simulink model "MRAS_IR2_Ld_Lq"  (R2019b)
settings: Solver=ode23tb  StartTime=0.0  StopTime=3  MaxStep=1e-5  RelTol=5e-4  EnableMultiTasking=on
libraries: powerlib x8, powerlib_meascontrol x2, simulink x1
settings Model: Creator=Алексей  LastModifiedBy=Len_comp
settings SolverCC: ZeroCrossControl=DisableAll  ZeroCrossAlgorithm=Adaptive
settings DataIOCC: SaveFormat=Array  SaveOutput=off  DSMLogging=off  SaveTime=off  ReturnWorkspaceOutputs=off
settings OptimizationCC: LifeSpan=inf
settings DebuggingCC: UnderspecifiedInitializationDetection=Classic  MergeDetectMultiDrivingBlocksExec=none  SolverPrmCheckMsg=warning  AllowSymbolicDim=off  SFUnexpectedBacktrackingDiag=warning  SFNoUnconditionalDefaultTransitionDiag=warning  SFExecutionAtInitializationDiag=none  ArithmeticOperatorsInVariantConditions=warning
settings HardwareCC: ProdBitPerPointer=32  ProdBitPerSizeT=32  ProdBitPerPtrDiffT=32  ProdLargestAtomicFloat=None  ProdIntDivRoundTo=Undefined  ProdEndianess=Unspecified  ProdWordSize=32  ProdHWDeviceType=32-bit Generic
settings ModelReferenceCC: PropagateSignalLabelsOutOfModel=off
settings SFSimCC: SimUseLocalCustomCode=off  CustomCodeUndefinedFunction=UseInterfaceOnly
settings RTWCC: RTWUseLocalCustomCode=off
settings CodeAppCC: StateflowObjectComments=on
settings GRTTargetCC: TargetLangStandard=C89/C90 (ANSI)  GeneratePreprocessorConditionals=Disable all
settings ConfigComp: CovMetricSettings=dw  CovHtmlReporting=on  CovSaveCumulativeToWorkspaceVar=on  CovSaveSingleToWorkspaceVar=on  CovExternalEMLEnable=off  CovSFcnEnable=off
settings SimscapeCC: SimscapeNormalizeSystem=off

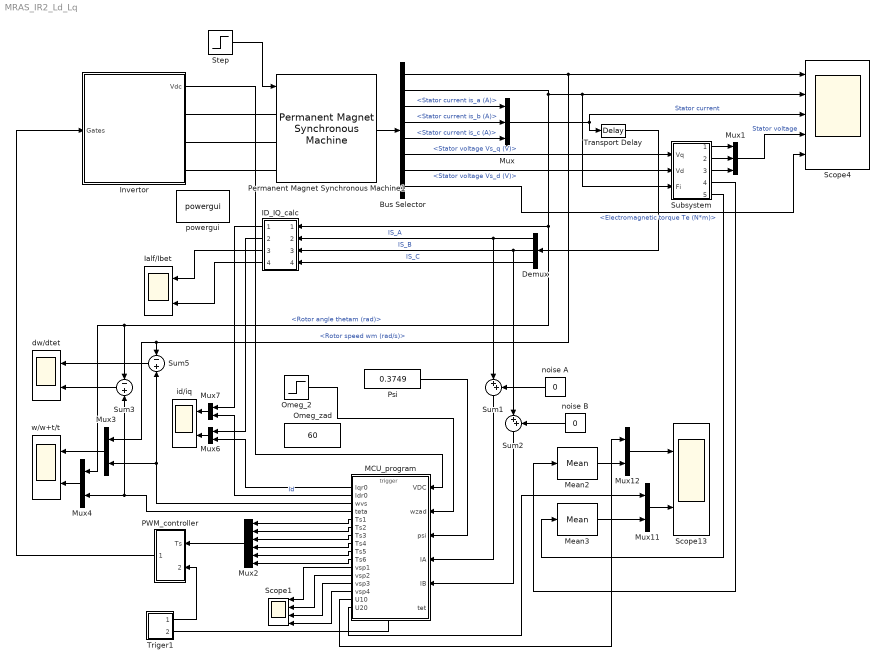
== system MRAS_IR2_Ld_Lq ==
  Bus Selector : BusSelector  OutputSignals=Rotor speed wm (rad/s),Rotor angle thetam (rad),Stator current is_a (A),Stator current is_b (A),Stator current is_c (A),Stator voltage Vs_q (V),Stator voltage Vs_d (V),Electromagnetic torque Te (N*m)
  Demux : Demux  Outputs=3
  ID_IQ_calc : Subsystem
  Ialf/Ibet : Scope  NumInputPorts=2
  Invertor : Subsystem
  MCU_program : MATLAB Function  TreatAsAtomicUnit=on
  Mean2 : powerlib_meascontrol/Measurements/Mean  Freq=10000  Vinit=0  Ts=0
      settings: SourceProductName=Simscape Electrical
  Mean3 : powerlib_meascontrol/Measurements/Mean  Freq=10000  Vinit=0  Ts=0
      settings: SourceProductName=Simscape Electrical
  Mux : Mux  Inputs=3
  Mux1 : Mux  Inputs=3
  Mux{3..4,6..7,11..12} (6 alike) : Mux  Inputs=2
  Mux2 : Mux  Inputs=6
  Omeg_2 : Step  Time=2.4  Before=60  After=100  SampleTime=0
  Omeg_zad : Constant  Value=60
  PWM_controller : Subsystem
  Permanent Magnet Synchronous Machine1 : powerlib/Machines/Permanent Magnet Synchronous Machine  NbPhases=3  FluxDistribution=Sinusoidal  RotorType=Salient-pole  MechanicalLoad=Torque Tm  PresetModel=No  ShowDetailedParameters=on  MeasurementBus=off  Resistance=13.75  Inductance=8.5e-3  dqInductances=[44e-3,39.8e-3]  La=40e-3  MachineConstant=Voltage Constant (V_peak L-L / krpm)  Flux=0.3749  VoltageCst=68  TorqueCst=0.56236  Flat=120  Mechanical=[2e-04 3e-03 1 0]  PolePairs=1  InitialConditions=[0,0, 0,0]  InitialConditions5ph=[0 0 0 0 0 0]  RefAngle=Aligned with phase A axis (original Park)  IterativeDiscreteModel=Trapezoidal non iterative  TsBlock=-1  TsPowergui=0
  Psi : Constant  Value=0.3749
  Scope1 : Scope  NumInputPorts=4
  Scope13 : Scope  NumInputPorts=2
  Scope4 : Scope  NumInputPorts=5
  Step : Step  Time=1.8  Before=0.02  After=0.07  SampleTime=0
  Subsystem : Subsystem
  Sum1 : Sum  Inputs=|++
  Sum2 : Sum  Inputs=|++
  Sum3 : Sum  Inputs=-+
  Sum5 : Sum  Inputs=-+
  Transport Delay : TransportDelay  DelayTime=5e-6
  Triger1 : Subsystem
  dw/dtet : Scope  NumInputPorts=2
  id/iq : Scope  NumInputPorts=2
  noise A : Constant  Value=0
  noise B : Constant  Value=0
  powergui : powerlib/powergui  Priority=1  SimulationMode=Continuous  SampleTime=50e-6  frequency=60  Iterations=50  frequencyindice=0  Pbase=100e6  ErrMax=1e-4  UnitsV=kV  UnitsW=MW  buscounter=0  FunctionMessages=off  echomessages=off  EnableUseOfTLC=off  CurrentSourceSwitches=on  DisableSnubberDevices=off  DisableRonSwitches=off  DisableVfSwitches=off  DisplayEquations=off  AutomaticDiscreteSolvers=off  SolverType=Tustin  Interpol=off  ExternalGateDelay=off  methode=off  Ts=0  x0status=blocks  SPID=off  SwTol=0  HookPort=off  NonlinearTolerance=1e-4  nMaxIteration=100  ContinueOnMaxIteration=off  RestoreLinks=warning  ResistiveCurrentMeasurement=off  Frange=[0:2:500]  Ylog=off  Xlog=on  ShowGrid=off  save=off  variable=ZData  structure=SD2  ZoomFFT=on  StartTime=0.7  cycles=10  DisplayStyle=4  fundamental=382  FreqAxis=off  MaxFrequency=50000  frequencyindicesteady=1  RmsSteady=1  display=off
      settings: SourceProductName=Simscape Electrical
  w/w+t/t : Scope  NumInputPorts=2
  wires:
  Demux/1 -> ID_IQ_calc/2(In2), Sum1/1  "IS_A"
  Demux/2 -> ID_IQ_calc/3(In3), Sum2/1  "IS_B"
  MCU_program/2(Idr0) -> Mux7/2  "Id"
  Omeg_2/1 -> MCU_program/2(wzad)
  Permanent Magnet Synchronous Machine1/1 -> Bus Selector/1
  Bus Selector/3 -> Mux/1  "<Stator current is_a (A)>"
  Bus Selector/4 -> Mux/2  "<Stator current is_b (A)>"
  Bus Selector/5 -> Mux/3  "<Stator current is_c (A)>"
  Bus Selector/6 -> Subsystem/1(Vq)  "<Stator voltage Vs_q (V)>"
  Bus Selector/7 -> Subsystem/2(Vd)  "<Stator voltage Vs_d (V)>"
  Subsystem/2(Out2) -> Mux1/2
  Subsystem/3(Out3) -> Mux1/3
  Subsystem/1(Out1) -> Mux1/1
  Mux/1 -> Scope4/3, Transport Delay/1  "Stator current"
  MCU_program/3(wvs) -> Mux3/2, Sum5/2
  Mux1/1 -> Scope4/4  "Stator voltage"
  Bus Selector/8 -> Scope4/5  "<Electromagnetic torque Te (N*m)>"
  Mux7/1 -> id/iq/1
  Mux6/1 -> id/iq/2
  Demux/3 -> ID_IQ_calc/4(In4)  "IS_C"
  Sum3/1 -> dw/dtet/2
  Sum5/1 -> dw/dtet/1
  MCU_program/4(teta) -> Mux4/2, Sum3/2
  ID_IQ_calc/1(Out1) -> Mux7/1
  ID_IQ_calc/2(Out2) -> Mux6/1
  Step/1 -> Permanent Magnet Synchronous Machine1/1
  MCU_program/5(Ts1) -> Mux2/1
  MCU_program/6(Ts2) -> Mux2/2
  MCU_program/7(Ts3) -> Mux2/3
  MCU_program/8(Ts4) -> Mux2/4
  MCU_program/9(Ts5) -> Mux2/5
  MCU_program/10(Ts6) -> Mux2/6
  Mux2/1 -> PWM_controller/1(Ts)
  Triger1/1(1) -> PWM_controller/2(pila)
  PWM_controller/1(Tss) -> Invertor/1(Gates)
  Mux3/1 -> w/w+t/t/1
  Mux4/1 -> w/w+t/t/2
  MCU_program/12(vsp2) -> Scope1/2
  MCU_program/13(vsp3) -> Scope1/3
  MCU_program/11(vsp1) -> Scope1/1
  Sum1/1 -> MCU_program/4(IA)
  Sum2/1 -> MCU_program/5(IB)
  Psi/1 -> MCU_program/3(psi)
  MCU_program/15(U10) -> Mux12/1
  Bus Selector/1 -> Scope4/1, Mux3/1, Sum5/1  "<Rotor speed wm (rad/s)>"
  Bus Selector/2 -> Mux4/1, Sum3/1, ID_IQ_calc/1(In1), Scope4/2, Subsystem/3(Fi)  "<Rotor angle thetam (rad)>"
  Triger1/2(2) -> MCU_program/Trigger
  MCU_program/16(U20) -> Mux11/1
  Mux12/1 -> Scope13/1
  Mux11/1 -> Scope13/2
  Mean3/1 -> Mux11/2
  Mean2/1 -> Mux12/2
  Invertor/1(Vdc) -> MCU_program/1(VDC)
  Subsystem/4(Out4) -> Mean2/1
  Subsystem/5(Out5) -> Mean3/1
  Transport Delay/1 -> Demux/1
  MCU_program/1(Iqr0) -> Mux6/2
  noise A/1 -> Sum1/2
  noise B/1 -> Sum2/2
  MCU_program/14(vsp4) -> Scope1/4
  ID_IQ_calc/3(Out3) -> Ialf/Ibet/1
  ID_IQ_calc/4(Out4) -> Ialf/Ibet/2
  connections:
  Permanent Magnet Synchronous Machine1/LConn1 -- Invertor/RConn1
  Invertor/RConn3 -- Permanent Magnet Synchronous Machine1/LConn3
  Permanent Magnet Synchronous Machine1/LConn2 -- Invertor/RConn2

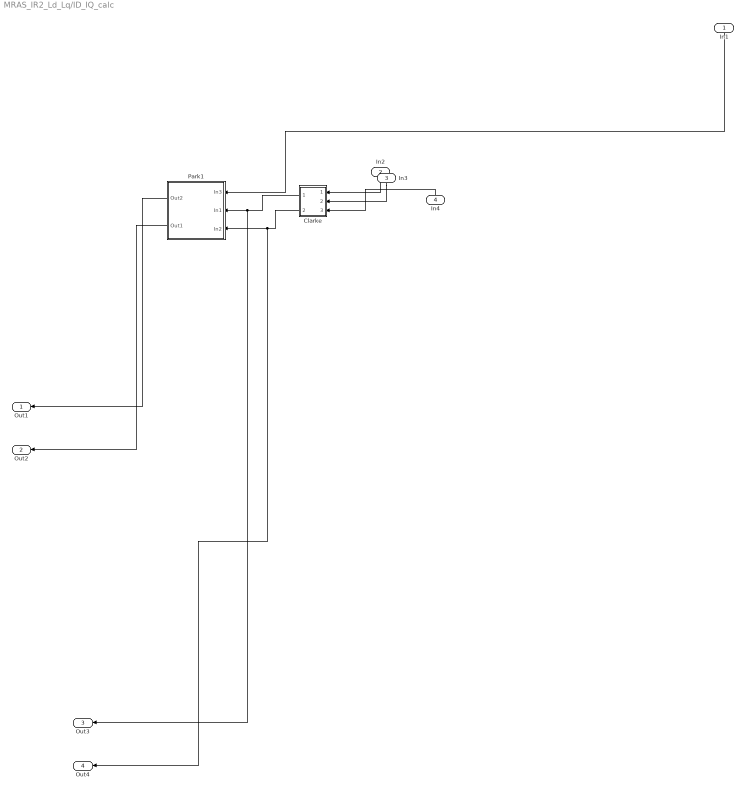
== system MRAS_IR2_Ld_Lq/ID_IQ_calc ==
  In1 : Inport
  In2 : Inport  Port=2
  In3 : Inport  Port=3
  In4 : Inport  Port=4
  Clarke : Subsystem
  Park1 : Subsystem
  Out1 : Outport
  Out2 : Outport  Port=2
  Out3 : Outport  Port=3
  Out4 : Outport  Port=4
  wires:
  Park1/2(Out1) -> Out2/1
  Park1/1(Out2) -> Out1/1
  In1/1 -> Park1/1(In3)
  In4/1 -> Clarke/3(In3)
  In2/1 -> Clarke/1(In1)
  In3/1 -> Clarke/2(In2)
  Clarke/2(Out1) -> Out4/1, Park1/3(In2)
  Clarke/1(Out2) -> Out3/1, Park1/2(In1)

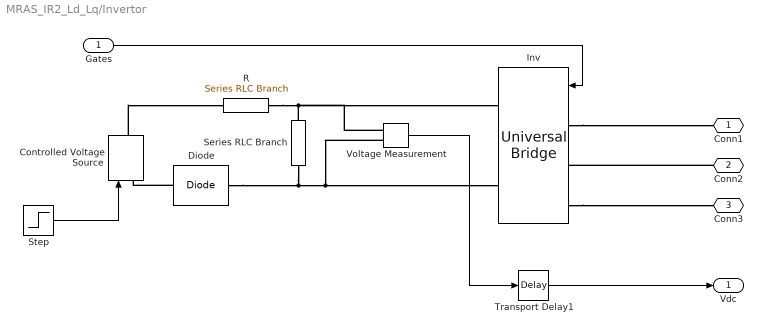
== system MRAS_IR2_Ld_Lq/Invertor ==
  Gates : Inport
  Controlled Voltage Source : powerlib/Electrical Sources/Controlled Voltage Source  Initialize=on  Source_Type=AC  Amplitude=0  Phase=0  Frequency=0  Measurements=None
      settings: SourceProductName=Simscape Electrical
  Diode : powerlib/Power Electronics/Diode  Ron=0.001  Lon=0  Vf=0.8  IC=0  UseSnubber=off  Rs=500  Cs=250e-9  Measurements=off
      settings: SourceProductName=Simscape Electrical
  Inv : powerlib/Power Electronics/Universal Bridge  Arms=3  SnubberResistance=1e5  SnubberCapacitance=inf  Device=IGBT / Diodes  Ron=1e-3  Lon=0  ForwardVoltages="[  3  3  ]"  ForwardVoltage=0  GTOparameters=[ 10e-6 , 20e-6 ]  IGBTparameters=[ 1e-7 , 2e-7 ]  Measurements=UAB UBC UCA UDC voltages  Measurements_2=None  converterType=Rectifier
      settings: SourceProductName=Simscape Electrical
  R : powerlib/Elements/Series RLC Branch  LConnTagsString=__new0  RConnTagsString=__new0  BranchType=R  Resistance=0.01  Inductance=1e-3  SetiL0=off  InitialCurrent=0  Capacitance=30e-6  Setx0=on  InitialVoltage=220  Measurements=None
      settings: SourceProductName=Simscape Electrical
  Series RLC Branch : powerlib/Elements/Series RLC Branch  LConnTagsString=__new0  RConnTagsString=__new0  BranchType=C  Resistance=1  Inductance=1e-3  SetiL0=off  InitialCurrent=0  Capacitance=30e-6  Setx0=on  InitialVoltage=20  Measurements=None
      settings: SourceProductName=Simscape Electrical
  Step : Step  Time=5.06  Before=150  After=300  SampleTime=0
  Transport Delay1 : TransportDelay  DelayTime=26e-6
  Voltage Measurement : powerlib/Measurements/Voltage Measurement  PhasorSimulation=off  OutputType=Complex  PSBequivalent=0
      settings: SourceProductName=Simscape Electrical
  Conn1 : PMIOPort  Side=Right
  Conn2 : PMIOPort  Port=2  Side=Right
  Conn3 : PMIOPort  Port=3  Side=Right
  Vdc : Outport
  wires:
  Gates/1 -> Inv/1
  Voltage Measurement/1 -> Transport Delay1/1
  Transport Delay1/1 -> Vdc/1
  Step/1 -> Controlled Voltage Source/1
  connections:
  Diode/LConn1 -- Series RLC Branch/RConn1 -- Voltage Measurement/LConn2 -- Inv/RConn2
  Series RLC Branch/LConn1 -- Voltage Measurement/LConn1 -- Inv/RConn1 -- R/LConn1
  Conn2/RConn1 -- Inv/LConn2
  Diode/RConn1 -- Controlled Voltage Source/LConn1
  Inv/LConn3 -- Conn3/RConn1
  Inv/LConn1 -- Conn1/RConn1
  Controlled Voltage Source/RConn1 -- R/RConn1

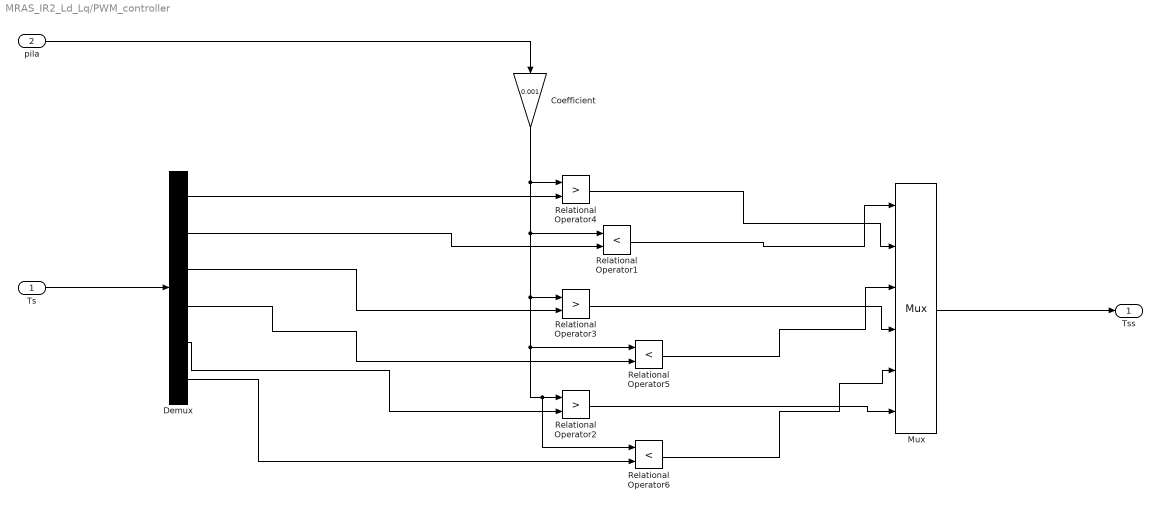
== system MRAS_IR2_Ld_Lq/PWM_controller ==
  Ts : Inport
  pila : Inport  Port=2
  Coefficient : Gain  Gain=0.001
  Demux : Demux  Outputs=6
  Mux : Mux  Inputs=6
  Relational Operator1 : RelationalOperator  Operator=<  OutDataTypeStr=boolean  RndMeth=Nearest
  Relational Operator2 : RelationalOperator  Operator=>  OutDataTypeStr=boolean  RndMeth=Nearest
  Relational Operator3 : RelationalOperator  Operator=>  OutDataTypeStr=boolean  RndMeth=Nearest
  Relational Operator4 : RelationalOperator  Operator=>  OutDataTypeStr=boolean  RndMeth=Nearest
  Relational Operator5 : RelationalOperator  Operator=<  OutDataTypeStr=boolean  RndMeth=Nearest
  Relational Operator6 : RelationalOperator  Operator=<  OutDataTypeStr=boolean  RndMeth=Nearest
  Tss : Outport
  wires:
  Relational Operator4/1 -> Mux/2
  Demux/3 -> Relational Operator3/2
  Demux/5 -> Relational Operator2/2
  Relational Operator3/1 -> Mux/4
  Relational Operator2/1 -> Mux/6
  Ts/1 -> Demux/1
  Coefficient/1 -> Relational Operator1/1, Relational Operator3/1, Relational Operator5/1, Relational Operator6/1, Relational Operator2/1, Relational Operator4/1
  Relational Operator1/1 -> Mux/1
  Relational Operator5/1 -> Mux/3
  Relational Operator6/1 -> Mux/5
  Demux/2 -> Relational Operator1/2
  Demux/4 -> Relational Operator5/2
  Demux/6 -> Relational Operator6/2
  Demux/1 -> Relational Operator4/2
  pila/1 -> Coefficient/1
  Mux/1 -> Tss/1

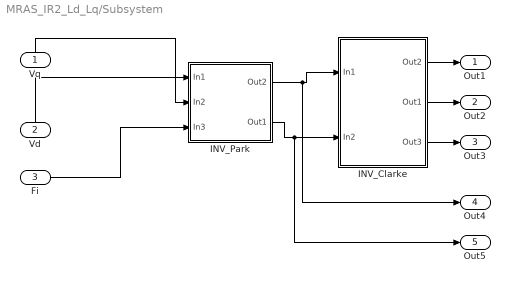
== system MRAS_IR2_Ld_Lq/Subsystem ==
  Vq : Inport
  Vd : Inport  Port=2
  Fi : Inport  Port=3
  INV_Clarke : Subsystem
  INV_Park : Subsystem
  Out1 : Outport
  Out2 : Outport  Port=2
  Out3 : Outport  Port=3
  Out4 : Outport  Port=4
  Out5 : Outport  Port=5
  wires:
  INV_Clarke/2(Out1) -> Out2/1
  INV_Park/1(Out2) -> Out4/1, INV_Clarke/1(In1)
  INV_Clarke/1(Out2) -> Out1/1
  INV_Park/2(Out1) -> Out5/1, INV_Clarke/2(In2)
  INV_Clarke/3(Out3) -> Out3/1
  Fi/1 -> INV_Park/3(In3)
  Vd/1 -> INV_Park/1(In1)
  Vq/1 -> INV_Park/2(In2)

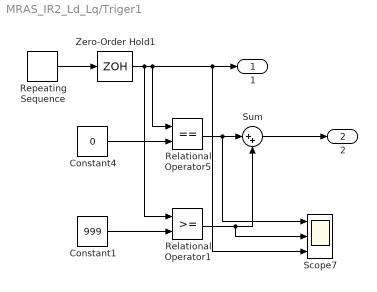
== system MRAS_IR2_Ld_Lq/Triger1 ==
  Constant1 : Constant  Value=999
  Constant4 : Constant  Value=0
  Relational Operator1 : RelationalOperator  OutDataTypeStr=boolean  RndMeth=Nearest
  Relational Operator5 : RelationalOperator  Operator===  OutDataTypeStr=boolean  RndMeth=Nearest
  Repeating Sequence : simulink/Sources/Repeating Sequence  rep_seq_t=[0 5e-5 10e-5]  rep_seq_y=[0 1000 0]
  Scope7 : Scope  NumInputPorts=3
  Sum : Sum  Inputs=|++
  Zero-Order Hold1 : ZeroOrderHold  SampleTime=25e-8
  1 : Outport
  2 : Outport  Port=2
  wires:
  Zero-Order Hold1/1 -> Relational Operator1/1, Relational Operator5/1, Scope7/3, 1/1
  Repeating Sequence/1 -> Zero-Order Hold1/1
  Constant4/1 -> Relational Operator5/2
  Sum/1 -> 2/1
  Constant1/1 -> Relational Operator1/2
  Relational Operator5/1 -> Scope7/1, Sum/1
  Relational Operator1/1 -> Scope7/2, Sum/2

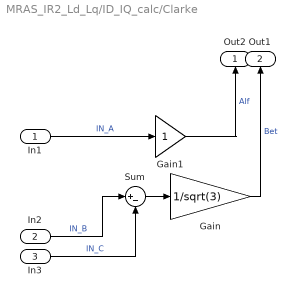
== system MRAS_IR2_Ld_Lq/ID_IQ_calc/Clarke ==
  In1 : Inport
  In2 : Inport  Port=2
  In3 : Inport  Port=3
  Gain : Gain  Gain=1/sqrt(3)
  Gain1 : Gain
  Sum : Sum  Inputs=|+-
  Out2 : Outport
  Out1 : Outport  Port=2
  wires:
  Gain/1 -> Out1/1  "Bet"
  In2/1 -> Sum/1  "IN_B"
  In1/1 -> Gain1/1  "IN_A"
  In3/1 -> Sum/2  "IN_C"
  Sum/1 -> Gain/1
  Gain1/1 -> Out2/1  "Alf"

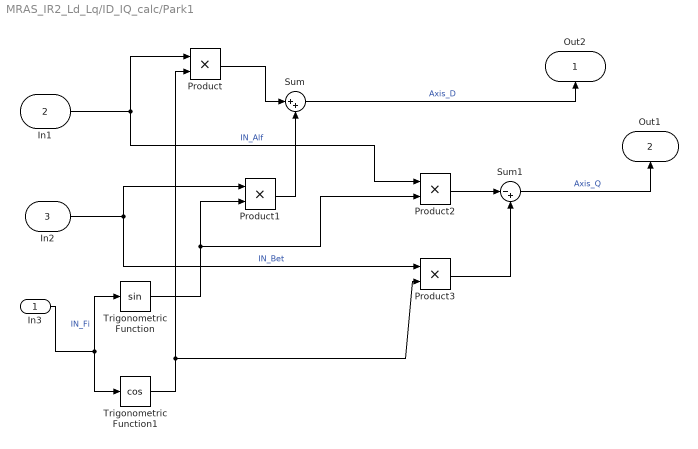
== system MRAS_IR2_Ld_Lq/ID_IQ_calc/Park1 ==
  In3 : Inport
  In1 : Inport  Port=2
  In2 : Inport  Port=3
  Product{,1..3} (4 alike) : Product
  Sum : Sum  Inputs=|++
  Sum1 : Sum  Inputs=|-+
  Trigonometric Function : Trigonometry
  Trigonometric Function1 : Trigonometry  Operator=cos
  Out2 : Outport
  Out1 : Outport  Port=2
  wires:
  Sum1/1 -> Out1/1  "Axis_Q"
  In2/1 -> Product1/1, Product3/1  "IN_Bet"
  In1/1 -> Product2/1, Product/1  "IN_Alf"
  Sum/1 -> Out2/1  "Axis_D"
  In3/1 -> Trigonometric Function1/1, Trigonometric Function/1  "IN_Fi"
  Trigonometric Function1/1 -> Product/2, Product3/2
  Trigonometric Function/1 -> Product2/2, Product1/2
  Product1/1 -> Sum/2
  Product/1 -> Sum/1
  Product2/1 -> Sum1/1
  Product3/1 -> Sum1/2

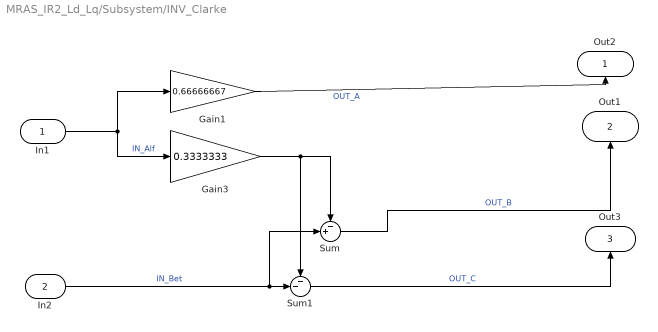
== system MRAS_IR2_Ld_Lq/Subsystem/INV_Clarke ==
  In1 : Inport
  In2 : Inport  Port=2
  Gain1 : Gain  Gain=0.66666667
  Gain3 : Gain  Gain=0.3333333
  Sum : Sum  Inputs=-+|
  Sum1 : Sum  Inputs=--|
  Out2 : Outport
  Out1 : Outport  Port=2
  Out3 : Outport  Port=3
  wires:
  Sum/1 -> Out1/1  "OUT_B"
  In2/1 -> Sum/2, Sum1/2  "IN_Bet"
  In1/1 -> Gain1/1, Gain3/1  "IN_Alf"
  Gain1/1 -> Out2/1  "OUT_A"
  Sum1/1 -> Out3/1  "OUT_C"
  Gain3/1 -> Sum1/1, Sum/1

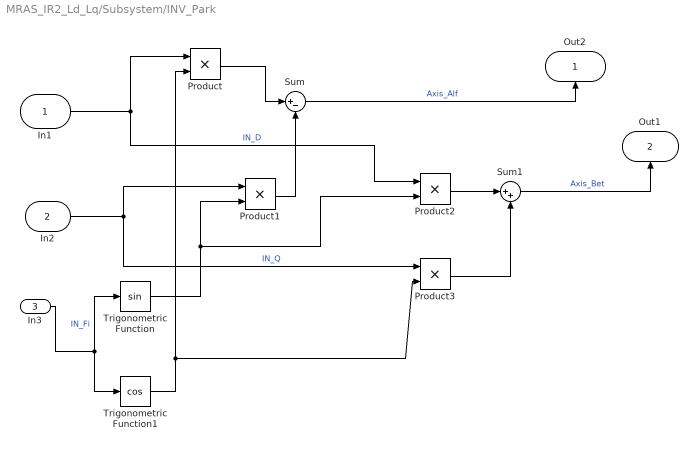
== system MRAS_IR2_Ld_Lq/Subsystem/INV_Park ==
  In1 : Inport
  In2 : Inport  Port=2
  In3 : Inport  Port=3
  Product{,1..3} (4 alike) : Product
  Sum : Sum  Inputs=|+-
  Sum1 : Sum  Inputs=|++
  Trigonometric Function : Trigonometry
  Trigonometric Function1 : Trigonometry  Operator=cos
  Out2 : Outport
  Out1 : Outport  Port=2
  wires:
  Sum1/1 -> Out1/1  "Axis_Bet"
  In2/1 -> Product1/1, Product3/1  "IN_Q"
  In1/1 -> Product2/1, Product/1  "IN_D"
  Sum/1 -> Out2/1  "Axis_Alf"
  In3/1 -> Trigonometric Function1/1, Trigonometric Function/1  "IN_Fi"
  Trigonometric Function1/1 -> Product/2, Product3/2
  Trigonometric Function/1 -> Product2/2, Product1/2
  Product1/1 -> Sum/2
  Product/1 -> Sum/1
  Product2/1 -> Sum1/1
  Product3/1 -> Sum1/2

== matlab function MRAS_IR2_Ld_Lq/MCU_program ==
  data: Iqr0 output; VDC input; wzad input; Idr0 output; psi input; wvs output; teta output; IA input; IB input; Ts1 output; Ts2 output; Ts3 output; Ts4 output; Ts5 output; Ts6 output; vsp1 output; vsp2 output; vsp3 output; vsp4 output; U10 output; U20 output; tet input
  events: trigger input RISING_EDGE_EVENT
function [Iqr0,Idr0,wvs,teta,Ts1,Ts2,Ts3,Ts4,Ts5,Ts6,vsp1,vsp2,vsp3,vsp4,U10,U20] = fcn(VDC,wzad,psi,IA,IB,tet)
%время 1/2 ШИМ периода
dt=50e-6;
%параметры машины
R=13.75;
Ld=42.4e-3;
Lq=37.81e-3;

%масимальный ток машины
cur_lim=0.8;
%Заданное значение тока по оси Дэ
Idzad=0;
%максимально допустимое значение момента на валу
T_max=cur_lim*psi/0.6667;

%Коэффициенты Пи-регулятора для МРАС
kint=15000;
kp=20;%.3;%16;


ktp=0.01;%0.02;
kti=0.350;%.075;

kuqp=185;
kuqi=17500;

kudp=285;
kudi=27500;


%Скорость при достижении которой переходим на МРАС 
wstart=20;
%Уголовое ускорение в разомкнутом режиме
eps=100;



persistent count1;
persistent count_w;
persistent Ialfa;
persistent Ibeta;
persistent wrez;
persistent wst;
persistent omeg;
persistent tew;
persistent tetm;
persistent wint;
persistent dId;
persistent dIq;
persistent Id; 
persistent Iq;
persistent Ua0; 
persistent Ub0;
persistent Uqint;
persistent Udint;
persistent start_fl;
persistent omega_fl;
persistent T_int;
persistent currentq;
persistent currentd;

%заполнение начальных значений static переменным (persistent здесь)
if isempty(count1)
    count1=0;
end ;
if isempty(count_w)
    count_w=0;
end ;


if isempty(wrez)
    wrez=0;
end ;

if isempty(wst)
    wst=0;
end ;

if isempty(omeg)
    omeg=0;
end ;
if isempty(tew)
    tew=-pi/2;
end ;

if isempty(tetm)
    tetm=0;
end ;

if isempty(wint)
    wint=0;
end ;

if isempty(Ua0)
    Ua0=0;
end ; 
if isempty(Ub0)
    Ub0=0;
end ;
if isempty(Id)
    Id=0;
end ;  
if isempty(Iq)
    Iq=0;
end ;
if isempty(Uqint)
    Uqint=0;
end ;
if isempty(Udint)
    Udint=0;
end ;
if isempty(start_fl)
    start_fl=0;
end ;
if isempty(omega_fl)
    omega_fl=0;
end ;
if isempty(T_int)
    T_int=0;
end ;
if isempty(currentq)
    currentq=0;
end ;
if isempty(currentd)
    currentd=0;
end ;
 
%------------------------------------------------------------------------------------------------------------
%Расчёт угла поворота через модель
%------------------------------------------------------------------------------------------------------------
%Преобразование Кларка
Ialfa=IA;
Ibeta=(2*IB+IA)/1.7320508;

 
Idr=Ialfa*cos(tet)+Ibeta*sin(tet);
Iqr=Ibeta*cos(tet)-Ialfa*sin(tet); 



  if(wst>=wstart)
    start_fl=1;
  end
  
elseif(start_fl==1)% если система находится в переходном реиме
  T_pr=0;
  count1=count1+1;
  if(count1>50)
  start_fl=2;
  wst=0;
  count1=0;
  end;
  tew=tew+wst*dt;
  torque=-1;
  cur_q=cur_lim;
  currentq=Iqr;
  currentd=Idr;
  tet=tew;
  Idr=Ialfa*cos(tet)+Ibeta*sin(tet);
  Iqr=Ibeta*cos(tet)-Ialfa*sin(tet); 

%------------------------------------------------------------------------------------------------------------
%если система в рабочем режиме
%------------------------------------------------------------------------------------------------------------
    
else
  count_w=count_w+1;
  wst=wst+wrez;
  if(count_w>=10)
      count_w=0;
      omeg=wst/10;
      wst=0;
  end;
%  omeg=wrez;
%  wst=wrez;
  if(omega_fl==0)
    if(currentd<0.01)
      omega_fl=1;
    end
    % определение поперечной составляющей тока, для требуемого момента
    cur_q=currentq;
    T_pr=cur_q*psi/0.6667;
    currentd=currentd*0.995;
    Idzad=currentd;
    tet=tetm;
    
    
    % если скорость приблизилась к требуемой, то стандартный ПИ алгоритм
  elseif(omega_fl==1)
    
    if(count1<200)
      count1=count1+1;
      cur_q=currentq;
      tet=tetm;
      T_pr=cur_q*psi/0.6667;
    else
      T_pr=(wzad-omeg)*ktp;
      tet=tetm;    
      cur_q=T_pr*0.6667/psi;
      currentq=currentq+0.0001*(cur_q-currentq);
      if(abs(cur_q-currentq)<0.01)
        omega_fl=2;   
      end;
      cur_q=currentq;
    end;
  else
    T_pr=(wzad-omeg)*ktp;
    if(T_pr>T_max)
        T_pr=T_max;
    elseif(T_pr<-T_max)
        T_pr=-T_max;
    end;
   % if(abs(wzad-omeg)<35)
      T_int=T_int+(wzad-omeg)*kti*dt;
    %end
    if(T_int+T_pr>T_max)
      T_int=T_max-T_pr;
    elseif(T_int<0)
        T_int=0;
    end;
      %формирование момента, требуемого на валу
    torque=T_pr+T_int;
    % определение поперечной составляющей тока, для требуемого момента
    cur_q=torque*0.6667/psi;
    if(cur_q>cur_lim) 
      cur_q=cur_lim;
    elseif (cur_q<0.01)
      cur_q=0.01;
    end
    tet=tetm;
  end
  
end;

%ПИ-регулятор для напряжения по оси Ку
diq=cur_q-Iqr;
Uqpr=diq*kuqp;
Uqint=Uqint+diq*kuqi*dt;

%ПИ-регулятор для напряжения по оси Дэ
did=Idzad-Idr;
Udpr=did*kudp;
Udint=Udint+did*kudi*dt;

Um=(2/3)*VDC/sqrt(Uqpr^2+Udpr^2);

if(Um<1)
  Uqpr=Uqpr*Um;
  Udpr=Udpr*Um;
end;

if((Uqpr+Uqint)>0.85*VDC)
  Uqint=0.85*VDC-Uqpr;
end;

if(sqrt((Uqpr+Uqint)^2+(Udpr+Udint)^2)>0.85*VDC)
  Udint=sqrt((0.85*VDC)^2-(Uqpr+Uqint)^2)-Udpr;
end;
if(Uqint<0)
  Uqint=0;
end;
if(Udint<0)
  Udint=0;
end;
  
U_q=Uqpr+Uqint;%+1.5*(L*Idr+psi)*wstart%wrez;                    %15.11 поменял omeg на wrez, интересно, как скажется на точности
U_d=Udpr+Udint;%-1.5*(wstart*Iqr*L);   %wrez      %15.11 поменял omeg на wrez, интересно, как скажется на точности

Ua0=U_d*cos(tet)-U_q*sin(tet);
Ub0=U_d*sin(tet)+U_q*cos(tet);

vrefa=sqrt(Ua0^2+Ub0^2);

vphase=acos(Ua0/vrefa)*sign(Ub0)+(sign(Ub0)-1)*(-pi);

if(vrefa>(2/3)*VDC)
  vrefa=(2/3)*VDC;
end
%вывод на осциллографы


teta=tetm;
wvs=wrez;


vsp1=T_pr;
vsp2=T_int;
vsp3=currentd;%wzad-omeg;
vsp4=omega_fl;
U10=Ua0;
U20=Ub0;


%алгоритм формирования векторной ШИМ  мертвым веменем dead [мкс]
dead=0;%0.75;
dead=dead/(dt*1e6);
a=vphase;
v2=vrefa*1.5;
if a>=0 && a<pi/3 
    n=1;
elseif  a>=pi/3 && a<2*pi/3 
    n=2;
elseif  a>=2*pi/3 && a<pi 
    n=3;
elseif  a>=pi && a<4*pi/3 
    n=4;
elseif  a>=4*pi/3 && a<5*pi/3 
    n=5;
else n=6;

end

a_cor=a-(n-1)*pi/3;

T1 = (v2/VDC)*sin(pi/3-a_cor)/sin(pi/3);
T2 = (v2/VDC)*sin(a_cor)/sin(pi/3);
T0=1-T1-T2;
Ta1=0; Ta3=0; Ta5=0; 
switch n
    case 1
        
        Ta1=T1+T2+T0/2;
        
        Ta3=T2+T0/2;
       
        Ta5=T0/2;
       
    case 2
        
        Ta1=T1+T0/2;
        
        Ta3=T1+T2+T0/2;
    
        Ta5=T0/2;       
        
    case 3
        
        Ta1=T0/2;
       
        Ta3=T1+T2+T0/2;
       
        Ta5=T2+T0/2;    
        
    case 4
        
        Ta1=T0/2;
       
        Ta3=T1+T0/2;
       
        Ta5=T1+T2+T0/2;   
       
    case 5
        
        Ta1=T2+T0/2;
        
        Ta3=T0/2;
        
        Ta5=T1+T2+T0/2;     
        
    case 6
        
        Ta1=T1+T2+T0/2;
        
        Ta3=T0/2;
     
        Ta5=T1+T0/2;    
        
end;


Ts1=(Ta1)+dead/2; 
Ts3=(Ta3)+dead/2; 
Ts5=(Ta5)+dead/2;
Ts2=(Ta1)-dead/2; 
Ts4=(Ta3)-dead/2; 
Ts6=(Ta5)-dead/2;

%{
if (IA>0) 
    Ts1=Ts1+dead/2;
    Ts2=Ts2+dead/2;
else
    Ts1=Ts1-dead/2;
    Ts2=Ts2-dead/2;           
end;
if (IB>0) 
    Ts3=Ts3+dead/2;
    Ts4=Ts4+dead/2;
else
    Ts3=Ts3-dead/2;
    Ts4=Ts4-dead/2; 
end;  
if ((-IA-IB)>0) 
    Ts5=Ts5+dead/2;
    Ts6=Ts6+dead/2;
else
    Ts5=Ts5-dead/2;
    Ts6=Ts6-dead/2;           
end;
%}

return;
